simulink model "uncompansated_design_motor_velocity"  (R2017b)
settings: Solver=FixedStepAuto  StartTime=0.0  StopTime=inf  FixedStep=0.05  RelTol=1e-3  EnableMultiTasking=on
values from neighbouring files (symbols this model uses):
  rp = 2*pi/(64*gr)    (= 0.00327249234749)    [CL_Constants_PID.m]
  Ts = 0.0625    [CL_Constants_PID.m]
libraries: arduinolib x2, THLlib x2, simulink x1
settings Model: ExtModeTrigDuration=2  Creator=sysad  LastModifiedBy=sysad
settings OptimizationCC: PassReuseOutputArgsThreshold=0  MaxStackSize=64
settings DebuggingCC: ParameterTunabilityLossMsg=error
settings HardwareCC: ProdBitPerInt=16  ProdBitPerPointer=16  ProdBitPerSizeT=16  ProdBitPerPtrDiffT=16  ProdLargestAtomicFloat=None  ProdWordSize=8  ProdHWDeviceType=Atmel->AVR  UseEmbeddedCoderFeatures=off
settings SFSimCC: MATLABDynamicMemAlloc=off
settings RTWCC: SystemTargetFile=ert.tlc  HardwareBoard=Arduino Uno  TLCOptions=-aInlineSetEventsForThisBaseRateFcn=TLC_FALSE -aSuppressMultiTaskScheduler=TLC_FALSE -aRateBasedStepFcn=1  TemplateMakefile=ert_default_tmf  GenerateReport=on  Toolchain=Arduino AVR  BuildConfiguration=Faster Runs  LaunchReport=on
settings CodeAppCC: ForceParamTrailComments=on  OperatorAnnotations=on
settings ERTTargetCC: ERTCustomFileBanners=off  SupportContinuousTime=on  SupportNonInlinedSFcns=on  RemoveResetFunc=off  SupportVariableSizeSignals=on  ModelStepFunctionPrototypeControlCompliant=off

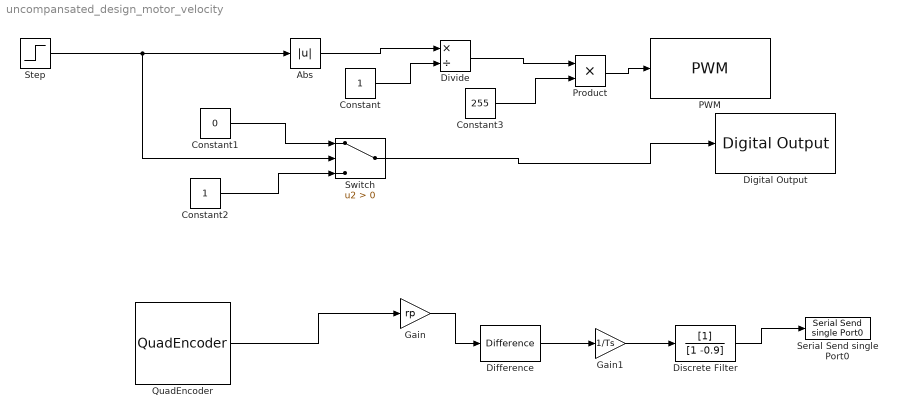
== system uncompansated_design_motor_velocity ==
  Abs : Abs
  Constant : Constant
  Constant1 : Constant  Value=0
  Constant2 : Constant
  Constant3 : Constant  Value=255
  Difference : simulink/Discrete/Difference  ICPrevInput=0.0  OutMin=[]  OutMax=[]  OutDataType=fixdt(1, 16)  OutScaling=2^-10  DoSatur=off
  Digital Output : arduinolib/Digital Output  pinNumber=4  blockPlatform=arduino
  Discrete Filter : DiscreteFilter  Denominator=[1 -0.9]
  Divide : Product  Inputs=*/
  Gain : Gain  Gain=rp
  Gain1 : Gain  Gain=1/Ts
  PWM : arduinolib/PWM  pinNumber=5  blockPlatform=arduino
  Product : Product
  QuadEncoder : THLlib/QuadEncoder
      settings: SourceProductName=Take Home Labs Arduino Support Package
  Serial Send single Port0 : THLlib/Serial Send single Port0
      settings: SourceProductName=Take Home Labs Arduino Support Package
  Step : Step  SampleTime=0
  Switch : Switch  Criteria=u2 > Threshold
  wires:
  Step/1 -> Switch/2, Abs/1
  Constant1/1 -> Switch/1
  Constant2/1 -> Switch/3
  Abs/1 -> Divide/1
  Constant/1 -> Divide/2
  Divide/1 -> Product/1
  Switch/1 -> Digital Output/1
  Product/1 -> PWM/1
  Discrete Filter/1 -> Serial Send single Port0/1
  Gain1/1 -> Discrete Filter/1
  Difference/1 -> Gain1/1
  Gain/1 -> Difference/1
  QuadEncoder/1 -> Gain/1
  Constant3/1 -> Product/2
